simulink model "EMC_no_gaze"  (R2015a)
settings: Solver=ode4  SolverMode=MultiTasking  StartTime=0.0  StopTime=inf  FixedStep=BKIN_STEP_TIME  RelTol=1e-3
StartFcn:
  |  warndlg('Dexterit-E models cannot run under simulation. Please compile your model and run it from within Dexterit-E.');set_param(bdroot,'SimulationCommand','stop')
model workspace (MAT data in the model file):
  BKIN_KINEMATIC_FRAME_SIZE = 400
  BKIN_STEP_TIME = 0.00025
  COLOR = 4
  COL_X = 1
  COL_Y = 2
  E_NO_EVENT = 0
  LOAD_X = 1
  LOAD_Y = 2
  MOVEMENT_DELAY = 3
  PATH_LENGTH = 1
  PATH_PERIOD = 2
  POST_TRIAL_DELAY = 4
  RADIUS = 3
  TRAJECTORY = 1
  TRAJECTORY_TYPE = 2
  TRIAL_END = 3
  TRIAL_MOVEMENT = 2
  TRIAL_RESET = 4
  TRIAL_START = 1
  X_POSITION = 1
  Y_POSITION = 2
  col_x = 1
  col_y = 2
  ANGULAR_THRESHOLD = 5
  GAZE_EXIT = 6
  START_REACHED = 7
  FIXATION_DURATION = 6
  TRACKING_TARGET_ROW = 7
  FEEDBACK_COLOR = 5
  CROSS_LOGICAL_RADIUS = 8
  DETECT_FIXATION = 8
  GAZE_IN_TARGET = 5
  START_STABILIZATION = 9
  HAND_IN_TARGET = 9
  BACKGROUND_LOAD = 10
  DIST_BETWEEN_TRAJ = 11
libraries: simulink x14, xpcrtudplib x12, xpcutilitieslib x10, xpcobsoletelib x8, ethercat x2, General x2, Video x2, KINARM_EP_loads x1, KINARM_general x1
(part 2 of 7)

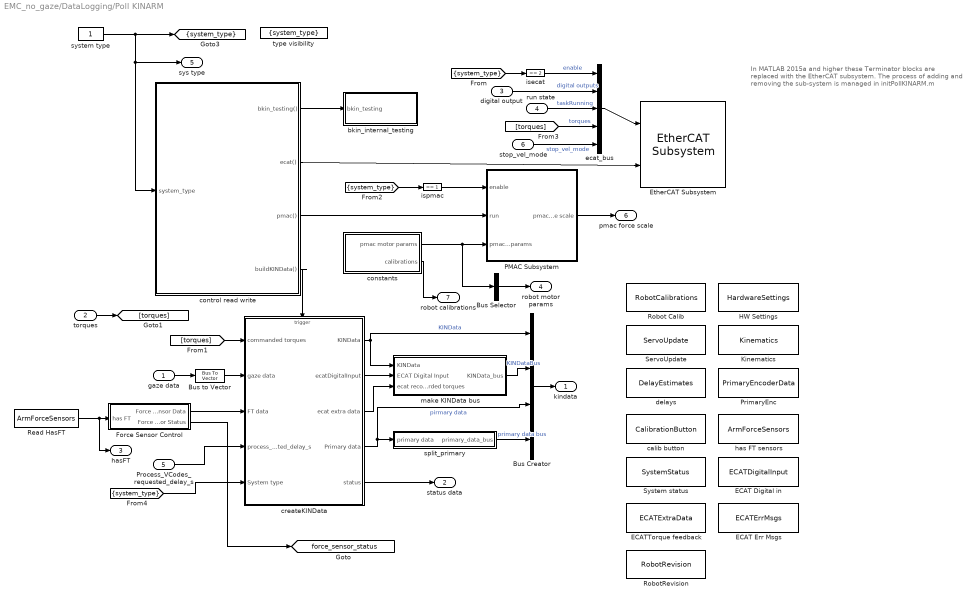
== system EMC_no_gaze/DataLogging/Poll KINARM ==
  note: In MATLAB 2015a and higher these Terminator blocks
      | are replaced with the EtherCAT subsystem. The process of
      | adding and removing the sub-system is managed in
      | initPollKINARM.m
  gaze data : Inport
  torques : Inport  Port=2
  digital output : Inport  Port=3
  run state : Inport  Port=4
  Process_VCodes_requested_delay_s : Inport  Port=5
  stop_vel_mode : Inport  Port=6
  Bus Creator : BusCreator
  Bus Selector : BusSelector  OutputSignals=robot1MotorParams,robot2MotorParams  OutputAsBus=on
  Bus to Vector : BusToVector
  ECAT Digital in : DataStoreMemory  DataStoreName=ECATDigitalInput  ReadBeforeWriteMsg=error  WriteAfterWriteMsg=warning  WriteAfterReadMsg=error  InitialValue=[0, 0, 0, 0, 0, 0, 0, 0]  OutDataTypeStr=uint32
  ECAT Err Msgs : DataStoreMemory  DataStoreName=ECATErrMsgs  ReadBeforeWriteMsg=error  WriteAfterWriteMsg=warning  WriteAfterReadMsg=error  InitialValue=zeros(4, 5)  OutDataTypeStr=double
  ECATTorque feedback : DataStoreMemory  DataStoreName=ECATExtraData  ReadBeforeWriteMsg=error  WriteAfterWriteMsg=warning  WriteAfterReadMsg=error  InitialValue=[0, 0, 0, 0, 0, 0, 0, 0, 0, 0]  OutDataTypeStr=double
  EtherCAT Subsystem : ethercat/EtherCAT Subsystem  SystemSampleTime=BKIN_STEP_TIME
  Force Sensor Control : Subsystem  TreatAsAtomicUnit=on
      settings: RTWSystemCode=Nonreusable function  RTWFileNameOpts=Use function name
  HW Settings : DataStoreMemory  DataStoreName=HardwareSettings  ReadBeforeWriteMsg=error  WriteAfterWriteMsg=warning  WriteAfterReadMsg=error  InitialValue=zeros(24, 1)  OutDataTypeStr=double
  Kinematics : DataStoreMemory  DataStoreName=Kinematics  ReadBeforeWriteMsg=error  WriteAfterWriteMsg=warning  WriteAfterReadMsg=error  InitialValue=zeros(20, 1)  OutDataTypeStr=double
  PMAC Subsystem : Subsystem
      settings: RTWSystemCode=Nonreusable function  RTWFileNameOpts=Use function name
  PrimaryEnc : DataStoreMemory  DataStoreName=PrimaryEncoderData  ReadBeforeWriteMsg=error  WriteAfterWriteMsg=warning  WriteAfterReadMsg=error  InitialValue=zeros(12, 1)  OutDataTypeStr=double
  Read HasFT : DataStoreRead  DataStoreName=ArmForceSensors  SampleTime=BKIN_STEP_TIME
  Robot Calib : DataStoreMemory  DataStoreName=RobotCalibrations  InitialValue=zeros(16, 1)  OutDataTypeStr=double
  RobotRevision : DataStoreMemory  DataStoreName=RobotRevision  ReadBeforeWriteMsg=error  WriteAfterWriteMsg=warning  WriteAfterReadMsg=error  InitialValue=[1, 1]  OutDataTypeStr=double
  ServoUpdate : DataStoreMemory  DataStoreName=ServoUpdate  ReadBeforeWriteMsg=error  WriteAfterWriteMsg=warning  WriteAfterReadMsg=error  OutDataTypeStr=uint32
  System status : DataStoreMemory  DataStoreName=SystemStatus  ReadBeforeWriteMsg=error  WriteAfterWriteMsg=warning  WriteAfterReadMsg=error  InitialValue=zeros(1, 7)  OutDataTypeStr=uint32
  bkin_internal_testing : Subsystem
  calib button : DataStoreMemory  DataStoreName=CalibrationButton  ReadBeforeWriteMsg=error  WriteAfterWriteMsg=warning  WriteAfterReadMsg=error  OutDataTypeStr=uint32
  constants : Subsystem
      settings: RTWSystemCode=Nonreusable function  RTWFileNameOpts=Use function name
  control read write : Stateflow chart  TreatAsAtomicUnit=on
  createKINData : Subsystem
      settings: RTWSystemCode=Nonreusable function  RTWFileNameOpts=Use function name
  delays : DataStoreMemory  DataStoreName=DelayEstimates  ReadBeforeWriteMsg=error  WriteAfterWriteMsg=warning  WriteAfterReadMsg=error  InitialValue=zeros(4, 1)  OutDataTypeStr=double
  ecat_bus : BusCreator  Inputs=5
  has FT sensors : DataStoreMemory  DataStoreName=ArmForceSensors  InitialValue=[0, 0]  OutDataTypeStr=double
  isecat : simulink/Logic and Bit Operations/Compare To Constant  relop===  const=2  OutDataTypeStr=boolean
  ispmac : simulink/Logic and Bit Operations/Compare To Constant  relop===  const=1  OutDataTypeStr=boolean
  make KINData bus : Subsystem
  split_primary : Subsystem
  system type : Constant
  type visibility : GotoTagVisibility  GotoTag=system_type
  kindata : Outport
  status data : Outport  Port=2
  hasFT : Outport  Port=3
  robot motor params : Outport  Port=4
  sys type : Outport  Port=5
  pmac force scale : Outport  Port=6
  robot calibrations : Outport  Port=7
  tag scope: force_sensor_status=global, system_type=scoped
  wires:
  control read write/2(ecat()) -> EtherCAT Subsystem/2
  ecat_bus/1 -> EtherCAT Subsystem/1
  stop_vel_mode/1 -> ecat_bus/5  "stop_vel_mode"
  Bus Selector/1 -> robot motor params/1
  Bus Creator/1 -> kindata/1
  Bus to Vector/1 -> createKINData/2(gaze data)
  constants/1(pmac motor params) -> Bus Selector/1, PMAC Subsystem/3(pmac robot params)
  createKINData/1(KINData) -> Bus Creator/1, make KINData bus/1(KINData)  "KINData"
  createKINData/4(Primary data) -> Bus Creator/3, split_primary/1(primary data)  "pirmary data"
  createKINData/5(status) -> status data/1
  gaze data/1 -> Bus to Vector/1
  Force Sensor Control/1(Force Sensor Data) -> createKINData/3(FT data)
  system type/1 -> [system_type], control read write/1(system_type), sys type/1
  control read write/1(bkin_testing()) -> bkin_internal_testing/1(bkin_testing)
  control read write/3(pmac()) -> PMAC Subsystem/2(run)
  control read write/4(buildKINData()) -> createKINData/Trigger
  [system_type] -> isecat/1
  [system_type] -> ispmac/1
  ispmac/1 -> PMAC Subsystem/1(enable)
  Read HasFT/1 -> hasFT/1, Force Sensor Control/1(has FT)
  make KINData bus/1(KINData_bus) -> Bus Creator/2  "KINDataBus"
  split_primary/1(primary_data_bus) -> Bus Creator/4  "primary data bus"
  PMAC Subsystem/1(pmac force scale) -> pmac force scale/1
  constants/2(calibrations) -> robot calibrations/1
  createKINData/2(ecatDigitalInput) -> make KINData bus/2(ECAT Digital Input)
  digital output/1 -> ecat_bus/2  "digital outputs"
  run state/1 -> ecat_bus/3  "taskRunning"
  isecat/1 -> ecat_bus/1  "enable"
  torques/1 -> [torques]
  [torques] -> createKINData/1(commanded torques)
  [torques] -> ecat_bus/4  "torques"
  createKINData/3(ecat extra data) -> make KINData bus/3(ecat recorded torques)
  Process_VCodes_requested_delay_s/1 -> createKINData/4(process_vcodes_requested_delay_s)
  Force Sensor Control/2(Force Sensor Status) -> [force_sensor_status]
  [system_type] -> createKINData/5(System type)

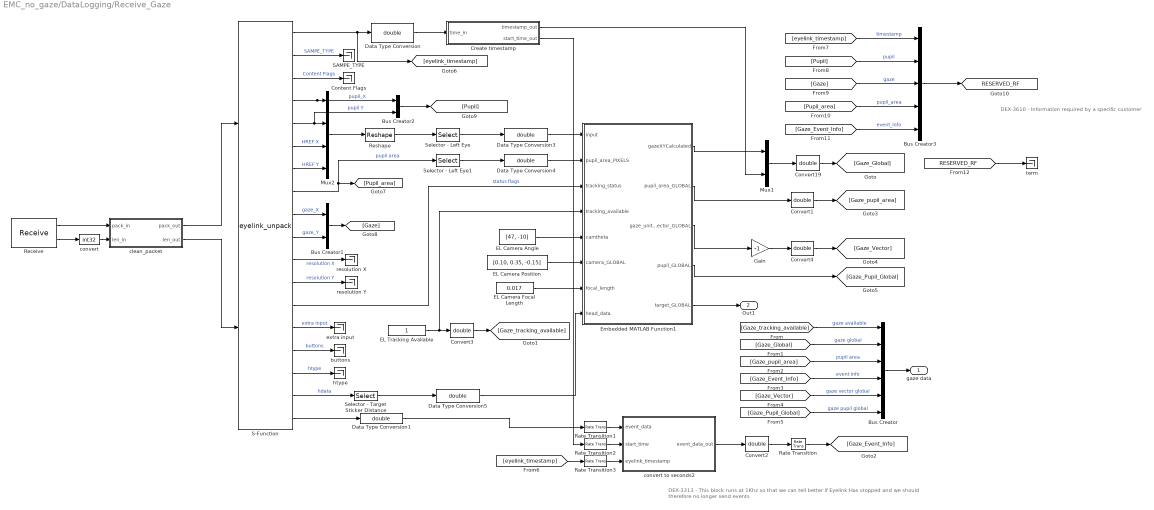
== system EMC_no_gaze/DataLogging/Receive_Gaze ==
  note: DEX-3610 - Information required by a specific customer
  note: DEX-3313 - This block runs at 1Khz so that we can tell better if Eyelink
      | Has stopped and we should therefore no longer send events
  Bus Creator : BusCreator  Inputs=6
  Bus Creator1 : BusCreator  Inputs=2
  Bus Creator2 : BusCreator  Inputs=2
  Bus Creator3 : BusCreator  Inputs=5
  Content Flags : Terminator
  Convert{1..4,19} (5 alike) : DataTypeConversion  OutDataTypeStr=double
  Create timestamp : MATLAB Function  TreatAsAtomicUnit=on
  Data Type Conversion{,1,3..5} (5 alike) : DataTypeConversion  OutDataTypeStr=double
  EL Camera Angle : Constant  Value=[47, -10]  VectorParams1D=off  OutDataTypeStr=double
  EL Camera Focal Length : Constant  Value=0.017  VectorParams1D=off  OutDataTypeStr=double
  EL Camera Position : Constant  Value=[0.10, 0.35, -0.15]  VectorParams1D=off  OutDataTypeStr=double
  EL Tracking Available : Constant  VectorParams1D=off  OutDataTypeStr=double
  Embedded MATLAB Function1 : MATLAB Function  TreatAsAtomicUnit=on
  Gain : Gain  Gain=-1
  Mux1 : Mux  Inputs=2
  Mux2 : Mux
  Rate Transition{,1..3} (4 alike) : RateTransition  Integrity=off
  Receive : xpcrtudplib/Legacy UDP/Receive   ipAddress=0.0.0.0  ipPort=4000  width=512  vblLen=on  sampletime=BKIN_STEP_TIME
  Reshape : Reshape  OutputDimensionality=Customize  OutputDimensions=[2,4]
  S-Function : S-Function  FunctionName=eyelink_unpack
  SAMPE_TYPE : Terminator
  Selector - Left Eye : Selector  NumberOfDimensions=2  InputPortWidth=3  IndexOptions=Index vector (dialog),Index vector (dialog)  Indices=1,-1  OutputSizes=1,1
  Selector - Left Eye1 : Selector
  Selector - Target Sticker Distance : Selector  Indices=1:3
  buttons : Terminator
  clean_packet : MATLAB Function  TreatAsAtomicUnit=on
  convert : DataTypeConversion  OutDataTypeStr=int32
  convert to seconds2 : MATLAB Function  TreatAsAtomicUnit=on  SystemSampleTime=0.001
  extra input : Terminator
  htype : Terminator
  resolution X : Terminator
  resolution Y : Terminator
  term : Terminator
  gaze data : Outport
  Out1 : Outport  Port=2
  tag scope: RESERVED_RF=global
  wires:
  Rate Transition3/1 -> convert to seconds2/3(eyelink_timestamp)
  Rate Transition2/1 -> convert to seconds2/2(start_time)
  Rate Transition1/1 -> convert to seconds2/1(event_data)
  [Gaze_Pupil_Global] -> Bus Creator/6  "gaze pupil global"
  Embedded MATLAB Function1/4(pupil_GLOBAL) -> [Gaze_Pupil_Global]
  Gain/1 -> Convert4/1
  Bus Creator/1 -> gaze data/1
  [Gaze_Event_Info] -> Bus Creator/4  "event info"
  [Gaze_pupil_area] -> Bus Creator/3  "pupil area"
  [Gaze_Global] -> Bus Creator/2  "gaze global"
  [Gaze_tracking_available] -> Bus Creator/1  "gaze available"
  EL Tracking Available/1 -> Embedded MATLAB Function1/4(tracking_available), Convert3/1
  EL Camera Position/1 -> Embedded MATLAB Function1/6(camera_GLOBAL)
  EL Camera Angle/1 -> Embedded MATLAB Function1/5(camtheta)
  Selector - Target Sticker Distance/1 -> Data Type Conversion5/1
  Selector - Left Eye/1 -> Data Type Conversion3/1
  Reshape/1 -> Selector - Left Eye/1
  Mux2/1 -> Reshape/1
  S-Function/7 -> Mux2/4  "HREF Y"
  S-Function/6 -> Mux2/3  "HREF X"
  S-Function/5 -> Bus Creator2/2, Mux2/2  "pupil Y"
  S-Function/4 -> Bus Creator2/1, Mux2/1  "pupil_X"
  Receive/2 -> convert/1
  S-Function/17 -> Selector - Target Sticker Distance/1  "hdata"
  S-Function/16 -> htype/1  "htype"
  S-Function/15 -> buttons/1  "buttons"
  S-Function/14 -> extra input/1  "extra input"
  S-Function/13 -> Embedded MATLAB Function1/3(tracking_status)  "status flags"
  S-Function/12 -> resolution Y/1  "resolution Y"
  S-Function/11 -> resolution X/1  "resolution X"
  S-Function/8 -> Selector - Left Eye1/1, [Pupil_area]  "pupil area"
  S-Function/3 -> Content Flags/1  "Content Flags"
  S-Function/2 -> SAMPE_TYPE/1  "SAMPE_TYPE"
  S-Function/9 -> Bus Creator1/1  "gaze_X"
  S-Function/10 -> Bus Creator1/2  "gaze_Y"
  Mux1/1 -> Convert19/1
  Embedded MATLAB Function1/1(gazeXYCalculated) -> Mux1/1
  Data Type Conversion/1 -> Create timestamp/1(time_in)
  S-Function/1 -> [eyelink_timestamp], Data Type Conversion/1
  S-Function/18 -> Data Type Conversion1/1
  Data Type Conversion1/1 -> Rate Transition1/1
  convert to seconds2/1(event_data_out) -> Convert2/1
  Create timestamp/2(start_time_out) -> Rate Transition2/1
  Data Type Conversion3/1 -> Embedded MATLAB Function1/1(input)
  Data Type Conversion5/1 -> Embedded MATLAB Function1/8(head_data)
  Embedded MATLAB Function1/2(pupil_area_GLOBAL) -> Convert1/1
  Data Type Conversion4/1 -> Embedded MATLAB Function1/2(pupil_area_PIXELS)
  EL Camera Focal Length/1 -> Embedded MATLAB Function1/7(focal_length)
  Selector - Left Eye1/1 -> Data Type Conversion4/1
  Receive/1 -> clean_packet/1(pack_in)
  convert/1 -> clean_packet/2(len_in)
  clean_packet/1(pack_out) -> S-Function/1
  clean_packet/2(len_out) -> S-Function/2
  Convert19/1 -> [Gaze_Global]
  Convert1/1 -> [Gaze_pupil_area]
  Convert2/1 -> Rate Transition/1
  Convert3/1 -> [Gaze_tracking_available]
  Convert4/1 -> [Gaze_Vector]
  Embedded MATLAB Function1/3(gaze_unit_vector_GLOBAL) -> Gain/1
  [Gaze_Vector] -> Bus Creator/5  "gaze vector global"
  Create timestamp/1(timestamp_out) -> Mux1/2
  Rate Transition/1 -> [Gaze_Event_Info]
  [eyelink_timestamp] -> Rate Transition3/1
  Bus Creator1/1 -> [Gaze]
  Bus Creator2/1 -> [Pupil]
  [Gaze_Event_Info] -> Bus Creator3/5  "event_info"
  [Pupil_area] -> Bus Creator3/4  "pupil_area"
  [Gaze] -> Bus Creator3/3  "gaze"
  [Pupil] -> Bus Creator3/2  "pupil"
  [eyelink_timestamp] -> Bus Creator3/1  "timestamp"
  Bus Creator3/1 -> [RESERVED_RF]
  [RESERVED_RF] -> term/1
  Embedded MATLAB Function1/5(target_GLOBAL) -> Out1/1

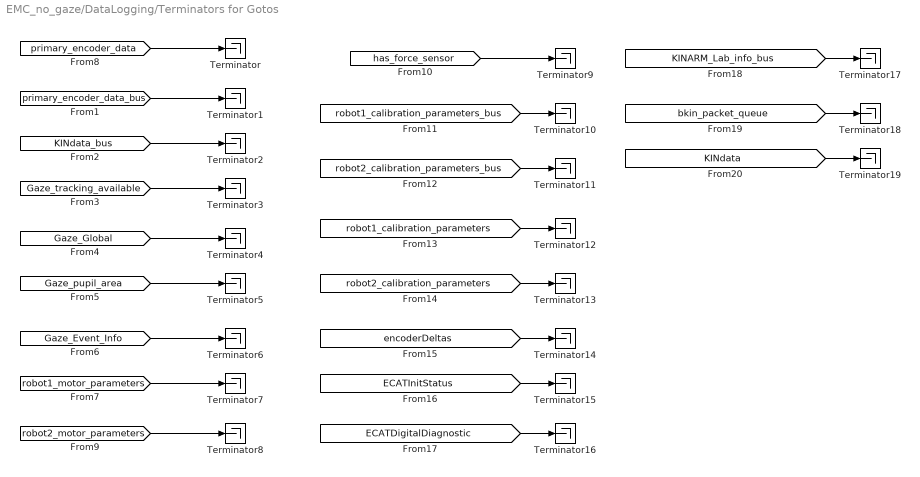
== system EMC_no_gaze/DataLogging/Terminators for Gotos ==
  Terminator{,1..19} (20 alike) : Terminator
  wires:
  [has_force_sensor] -> Terminator9/1
  [robot2_motor_parameters] -> Terminator8/1
  [robot1_motor_parameters] -> Terminator7/1
  [Gaze_Event_Info] -> Terminator6/1
  [Gaze_pupil_area] -> Terminator5/1
  [Gaze_Global] -> Terminator4/1
  [Gaze_tracking_available] -> Terminator3/1
  [KINdata_bus] -> Terminator2/1
  [primary_encoder_data_bus] -> Terminator1/1
  [primary_encoder_data] -> Terminator/1
  [robot1_calibration_parameters_bus] -> Terminator10/1
  [robot2_calibration_parameters_bus] -> Terminator11/1
  [robot1_calibration_parameters] -> Terminator12/1
  [robot2_calibration_parameters] -> Terminator13/1
  [encoderDeltas] -> Terminator14/1
  [ECATInitStatus] -> Terminator15/1
  [ECATDigitalDiagnostic] -> Terminator16/1
  [KINARM_Lab_info_bus] -> Terminator17/1
  [bkin_packet_queue] -> Terminator18/1
  [KINdata] -> Terminator19/1

== system EMC_no_gaze/DataLogging/apply loads ==
  system_type : Inport
  torques : Inport  Port=2
  pmac force scale : Inport  Port=3
  motor params : Inport  Port=4
  Bus Selector3 : BusSelector  OutputSignals=robot1MotorParams,robot2MotorParams
  EtherCAT Apply Loads : ethercat/ECAT Apply Loads
  apply pmac loads : Subsystem
      settings: RTWSystemCode=Nonreusable function  RTWFileNameOpts=Use function name
  isecat : simulink/Logic and Bit Operations/Compare To Constant  relop===  const=2  OutDataTypeStr=boolean
  isecat1 : simulink/Logic and Bit Operations/Compare To Constant  relop===  const=1  OutDataTypeStr=boolean
  verify NaN : MATLAB Function  TreatAsAtomicUnit=on
  wires:
  [torques] -> EtherCAT Apply Loads/1
  isecat/1 -> EtherCAT Apply Loads/Enable
  Bus Selector3/2 -> apply pmac loads/4(Robot 2 motor parms)  "<robot2MotorParams>"
  Bus Selector3/1 -> apply pmac loads/3(Robot 1 motor parms)  "<robot1MotorParams>"
  pmac force scale/1 -> apply pmac loads/1(Force scale)
  motor params/1 -> Bus Selector3/1
  [system_type] -> isecat1/1
  isecat1/1 -> apply pmac loads/Enable
  [system_type] -> isecat/1
  torques/1 -> verify NaN/1(torques_in)
  [torques] -> apply pmac loads/2(Torques)
  system_type/1 -> [system_type]
  verify NaN/1(torques_out) -> [torques]

== system EMC_no_gaze/DataLogging/compare encoders ==
  Bus Selector4 : BusSelector  OutputSignals=Robot1.a1_link_angles,Robot2.a2_link_angles
  Bus Selector5 : BusSelector  OutputSignals=robot1.a1_link_angles,robot2.a2_link_angles
  Mux : Mux  Inputs=2
  Mux1 : Mux  Inputs=2
  delta : MATLAB Function  TreatAsAtomicUnit=on
  encoder deltas : Outport
  wires:
  [KINdata_bus] -> Bus Selector4/1
  [primary_encoder_data_bus] -> Bus Selector5/1
  Bus Selector4/1 -> Mux/1  "<a1_link_angles>"
  Bus Selector4/2 -> Mux/2  "<a2_link_angles>"
  Bus Selector5/1 -> Mux1/1  "<a1_link_angles>"
  Bus Selector5/2 -> Mux1/2  "<a2_link_angles>"
  Mux/1 -> delta/1(secondaryEncAngles)
  Mux1/1 -> delta/2(primaryEncAngles)
  delta/1(deltas) -> encoder deltas/1

== system EMC_no_gaze/DataLogging/create_lab_info ==
  Bus Creator3 : BusCreator  Inputs=7
  Subsystem : Subsystem
  arm_count : Constant  Value=0
  fp1_present : Constant  Value=0
  fp2_present : Constant  Value=0
  gaze_tracker_present : Constant  Value=0
  robot_lift_present : Constant  Value=0
  tag scope: KINARM_Lab_info_bus=global
  wires:
  fp1_present/1 -> Bus Creator3/5  "has_force_plate_1"
  Bus Creator3/1 -> [KINARM_Lab_info_bus]
  Subsystem/2(robot_2_info) -> Bus Creator3/3  "robot_2"
  Subsystem/1(robot_1_info) -> Bus Creator3/2  "robot_1"
  robot_lift_present/1 -> Bus Creator3/7  "has_robot_lift"
  gaze_tracker_present/1 -> Bus Creator3/4  "has_gaze_tracker"
  arm_count/1 -> Bus Creator3/1  "robot_count"
  fp2_present/1 -> Bus Creator3/6  "has_force_plate_2"

== system EMC_no_gaze/DataLogging/gaze gotos ==
  In1 : Inport
  Bus Selector : BusSelector  OutputSignals=gaze available,gaze global,pupil area,event info,gaze vector global,gaze pupil global
  tag scope: Gaze_Event_Info=global, Gaze_Global=global, Gaze_Pupil_Global=global, Gaze_Vector_Global=global, Gaze_pupil_area=global, Gaze_tracking_available=global
  wires:
  Bus Selector/5 -> [Gaze_Vector_Global]  "<gaze vector global>"
  Bus Selector/6 -> [Gaze_Pupil_Global]  "<gaze pupil global>"
  Bus Selector/4 -> [Gaze_Event_Info]  "<event info>"
  Bus Selector/3 -> [Gaze_pupil_area]  "<pupil area>"
  Bus Selector/2 -> [Gaze_Global]  "<gaze global>"
  Bus Selector/1 -> [Gaze_tracking_available]  "<gaze available>"
  In1/1 -> Bus Selector/1

== system EMC_no_gaze/DataLogging/kindata gotos ==
  In1 : Inport
  Bus Selector1 : BusSelector  OutputSignals=KINData,KINDataBus,pirmary data,primary data bus
  tag scope: KINdata=global, KINdata_bus=global, primary_encoder_data=global, primary_encoder_data_bus=global
  wires:
  Bus Selector1/4 -> [primary_encoder_data_bus]  "<primary data bus>"
  Bus Selector1/3 -> [primary_encoder_data]  "<pirmary data>"
  Bus Selector1/2 -> [KINdata_bus]  "<KINDataBus>"
  Bus Selector1/1 -> [KINdata]  "<KINData>"
  In1/1 -> Bus Selector1/1

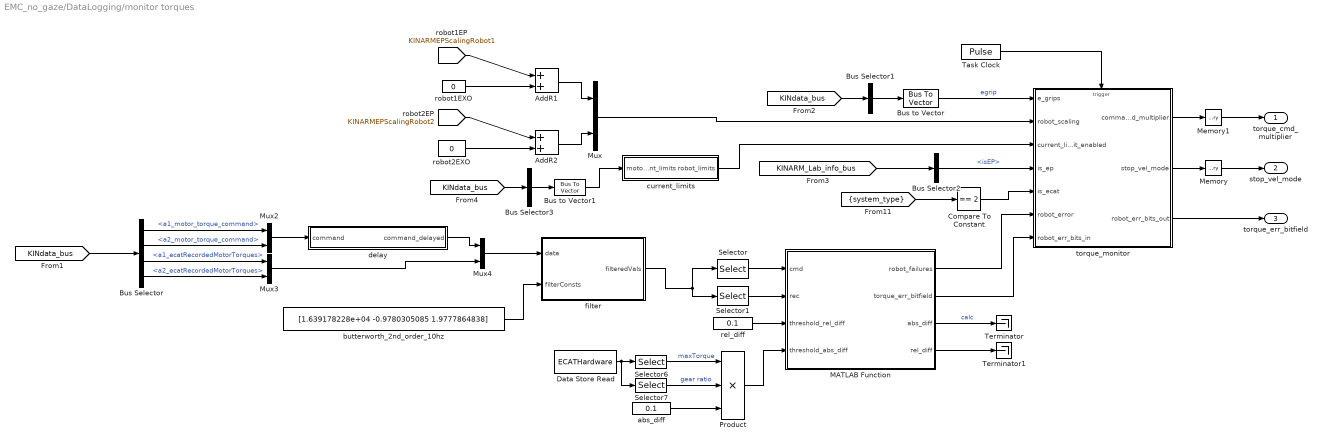
== system EMC_no_gaze/DataLogging/monitor torques ==
  AddR1 : Sum
  AddR2 : Sum
  Bus Selector : BusSelector  OutputSignals=Robot1.a1_motor_torque_command,Robot2.a2_motor_torque_command,Robot1.a1_ecatRecordedMotorTorques,Robot2.a2_ecatRecordedMotorTorques
  Bus Selector1 : BusSelector  OutputSignals=Robot1.a1_ep_grip_sensor,Robot2.a2_ep_grip_sensor  OutputAsBus=on
  Bus Selector2 : BusSelector  OutputSignals=robot_1.isEP
  Bus Selector3 : BusSelector  OutputSignals=Robot1.a1_ecatCurrentLimitEnabled,Robot2.a2_ecatCurrentLimitEnabled  OutputAsBus=on
  Bus to Vector : BusToVector
  Bus to Vector1 : BusToVector
  Compare To Constant : simulink/Logic and Bit Operations/Compare To Constant  relop===  const=2  OutDataTypeStr=boolean
  Data Store Read : DataStoreRead  DataStoreName=ECATHardware  SampleTime=BKIN_STEP_TIME
  MATLAB Function : MATLAB Function  TreatAsAtomicUnit=on
  Memory : Memory
  Memory1 : Memory
  Mux{,2..4} (4 alike) : Mux  Inputs=2
  Product : Product  Inputs=3
  Selector : Selector  Indices=[1:4]
  Selector1 : Selector  Indices=[5:8]
  Selector6 : Selector  Indices=[1:4]
  Selector7 : Selector  Indices=[5:8]
  Task Clock : DiscretePulseGenerator  PulseType=Time based  Period=.001  PulseWidth=50  SampleTime=0.0005
  Terminator : Terminator
  Terminator1 : Terminator
  abs_diff : Constant  Value=0.1
  butterworth_2nd_order_10hz : Constant  Value=[1.639178228e+04 -0.9780305085 1.9777864838]
  current_limits : MATLAB Function  TreatAsAtomicUnit=on  SystemSampleTime=BKIN_STEP_TIME
  delay : Subsystem
  filter : MATLAB Function  TreatAsAtomicUnit=on  SystemSampleTime=BKIN_STEP_TIME
  rel_diff : Constant  Value=0.1
  robot1EXO : Constant  Value=0
  robot2EXO : Constant  Value=0
  torque_monitor : Stateflow chart  TreatAsAtomicUnit=on
  torque_cmd_multiplier : Outport
  stop_vel_mode : Outport  Port=2
  torque_err_bitfield : Outport  Port=3
  wires:
  MATLAB Function/4(rel_diff) -> Terminator1/1
  MATLAB Function/3(abs_diff) -> Terminator/1  "calc"
  butterworth_2nd_order_10hz/1 -> filter/2(filterConsts)
  Mux4/1 -> filter/1(data)
  Memory/1 -> stop_vel_mode/1
  Memory1/1 -> torque_cmd_multiplier/1
  Bus Selector2/1 -> torque_monitor/4(is_ep)  "<isEP>"
  [system_type] -> Compare To Constant/1
  [KINARM_Lab_info_bus] -> Bus Selector2/1
  Bus to Vector/1 -> torque_monitor/1(e_grips)  "egrip"
  Bus Selector1/1 -> Bus to Vector/1
  [KINdata_bus] -> Bus Selector1/1
  MATLAB Function/1(robot_failures) -> torque_monitor/6(robot_error)
  Selector1/1 -> MATLAB Function/2(rec)
  Selector/1 -> MATLAB Function/1(cmd)
  filter/1(filteredVals) -> Selector/1, Selector1/1
  Mux3/1 -> Mux4/2
  delay/1(command_delayed) -> Mux4/1
  Mux2/1 -> delay/1(command)
  Bus Selector/3 -> Mux3/1  "<a1_ecatRecordedMotorTorques>"
  Bus Selector/4 -> Mux3/2  "<a2_ecatRecordedMotorTorques>"
  Bus Selector/2 -> Mux2/2  "<a2_motor_torque_command>"
  Bus Selector/1 -> Mux2/1  "<a1_motor_torque_command>"
  [KINdata_bus] -> Bus Selector/1
  Compare To Constant/1 -> torque_monitor/5(is_ecat)
  Task Clock/1 -> torque_monitor/Trigger
  torque_monitor/2(stop_vel_mode) -> Memory/1
  torque_monitor/1(command_multiplier) -> Memory1/1
  [KINdata_bus] -> Bus Selector3/1
  AddR1/1 -> Mux/1
  AddR2/1 -> Mux/2
  Bus Selector3/1 -> Bus to Vector1/1
  Mux/1 -> torque_monitor/2(robot_scaling)
  MATLAB Function/2(torque_err_bitfield) -> torque_monitor/7(robot_err_bits_in)
  torque_monitor/3(robot_err_bits_out) -> torque_err_bitfield/1
  Data Store Read/1 -> Selector7/1, Selector6/1
  Selector6/1 -> Product/1  "maxTorque"
  Product/1 -> MATLAB Function/4(threshold_abs_diff)
  Selector7/1 -> Product/2  "gear ratio"
  abs_diff/1 -> Product/3
  rel_diff/1 -> MATLAB Function/3(threshold_rel_diff)
  current_limits/1(robot_limits) -> torque_monitor/3(current_limit_enabled)
  Bus to Vector1/1 -> current_limits/1(motor_current_limits)
  robot1EXO/1 -> AddR1/2
  robot2EXO/1 -> AddR2/2
  [KINARMEPScalingRobot1] -> AddR1/1
  [KINARMEPScalingRobot2] -> AddR2/1

== system EMC_no_gaze/DataLogging/motor gotos ==
  In1 : Inport
  Bus Selector2 : BusSelector  OutputSignals=robot1MotorParams,robot2MotorParams
  tag scope: robot1_motor_parameters=global, robot2_motor_parameters=global
  wires:
  Bus Selector2/2 -> [robot2_motor_parameters]  "<robot2MotorParams>"
  Bus Selector2/1 -> [robot1_motor_parameters]  "<robot1MotorParams>"
  In1/1 -> Bus Selector2/1

== system EMC_no_gaze/DataLogging/robot gotos ==
  In1 : Inport
  Bus Selector3 : BusSelector  OutputSignals=robot1 calibration params,robot2 calibration params
  Bus to Vector : BusToVector
  Bus to Vector1 : BusToVector
  tag scope: robot1_calibration_parameters=global, robot1_calibration_parameters_bus=global, robot2_calibration_parameters=global, robot2_calibration_parameters_bus=global
  wires:
  Bus Selector3/1 -> [robot1_calibration_parameters_bus], Bus to Vector/1  "<robot1 calibration params>"
  Bus Selector3/2 -> [robot2_calibration_parameters_bus], Bus to Vector1/1  "<robot2 calibration params>"
  Bus to Vector/1 -> [robot1_calibration_parameters]
  Bus to Vector1/1 -> [robot2_calibration_parameters]
  In1/1 -> Bus Selector3/1

== system EMC_no_gaze/KINARM_EP_Apply_Loads/detect motor state ==
  Bus Selector1 : BusSelector  OutputSignals=R1Info.isECAT
  Bus Selector2 : BusSelector  OutputSignals=Robot1.a1_motor_status,Robot1.a1_ep_grip_sensor
  MATLAB Function : MATLAB Function  TreatAsAtomicUnit=on
  motors enabled : Outport
  wires:
  Bus Selector2/2 -> MATLAB Function/2(grip_sensor)  "<a1_ep_grip_sensor>"
  [robot1_motor_parameters] -> Bus Selector1/1
  Bus Selector2/1 -> MATLAB Function/1(motor_status)  "<a1_motor_status>"
  [KINdata_bus] -> Bus Selector2/1
  Bus Selector1/1 -> MATLAB Function/3(is_ecat)  "<isECAT>"
  MATLAB Function/1(motors_enabled) -> motors enabled/1

== system EMC_no_gaze/KINARM_EP_Apply_Loads/detect motor state1 ==
  Bus Selector1 : BusSelector  OutputSignals=R2Info.isECAT
  Bus Selector2 : BusSelector  OutputSignals=Robot2.a2_motor_status,Robot2.a2_ep_grip_sensor
  MATLAB Function : MATLAB Function  TreatAsAtomicUnit=on
  motors enabled : Outport
  wires:
  Bus Selector2/2 -> MATLAB Function/2(grip_sensor)  "<a2_ep_grip_sensor>"
  [robot2_motor_parameters] -> Bus Selector1/1
  Bus Selector2/1 -> MATLAB Function/1(motor_status)  "<a2_motor_status>"
  [KINdata_bus] -> Bus Selector2/1
  Bus Selector1/1 -> MATLAB Function/3(is_ecat)  "<isECAT>"
  MATLAB Function/1(motors_enabled) -> motors enabled/1

== system EMC_no_gaze/DataLogging/Create KINARM Data Subsystem/gaze_data ==
  Mux : Mux  Inputs=5
  gaze_channels : Outport
  wires:
  [Gaze_Global] -> Mux/1
  Mux/1 -> gaze_channels/1
  [Gaze_pupil_area] -> Mux/2
  [Gaze_Vector_Global] -> Mux/3
  [Gaze_Event_Info] -> Mux/5
  [Gaze_Pupil_Global] -> Mux/4

== system EMC_no_gaze/DataLogging/Create KINARM Data Subsystem/select KINData ==
  Bus Selector : BusSelector  OutputSignals=Robot1.a1_link_angles,Robot1.a1_link_velocities,Robot1.a1_link_accelerations,Robot1.a1_hand_position,Robot1.a1_motor_torque_command,Robot1.a1_force_sensor_force_xyz,Robot1.a1_force_sensor_torque_xyz,Robot1.a1_force_sensor_timestamp,Robot1.a1_ecatRecordedMotorTorques,Robot2.a2_link_angles,Robot2.a2_link_velocities,Robot2.a2_link_accelerations,Robot2.a2_hand_position,Robot2.a2_motor_torque_command,Robot2.a2_force_sensor_force_xyz,Robot2.a2_force_sensor_torque_xyz,Robot2.a2_force_sensor_timestamp,Robot2.a2_ecatRecordedMotorTorques,Robot1.a1_force_sensor_status,Robot2.a2_force_sensor_status
  Demux : Demux  Outputs=2
  MATLAB Function : MATLAB Function  TreatAsAtomicUnit=on
  Mux : Mux  Inputs=8
  Mux1 : Mux  Inputs=9
  Mux2 : Mux  Inputs=5
  Mux3 : Mux  Inputs=2
  Out1 : Outport
  wires:
  [KINdata_bus] -> Bus Selector/1
  Bus Selector/1 -> Mux/1  "<a1_link_angles>"
  Bus Selector/2 -> Mux/2  "<a1_link_velocities>"
  Bus Selector/3 -> Mux/3  "<a1_link_accelerations>"
  Bus Selector/4 -> Mux/4  "<a1_hand_position>"
  Bus Selector/5 -> Mux/5  "<a1_motor_torque_command>"
  Bus Selector/6 -> Mux/6  "<a1_force_sensor_force_xyz>"
  Bus Selector/7 -> Mux/7  "<a1_force_sensor_torque_xyz>"
  Bus Selector/8 -> Mux/8  "<a1_force_sensor_timestamp>"
  Bus Selector/9 -> Mux1/1  "<a1_ecatRecordedMotorTorques>"
  Bus Selector/10 -> Mux1/2  "<a2_link_angles>"
  Bus Selector/11 -> Mux1/3  "<a2_link_velocities>"
  Bus Selector/12 -> Mux1/4  "<a2_link_accelerations>"
  Bus Selector/13 -> Mux1/5  "<a2_hand_position>"
  Bus Selector/14 -> Mux1/6  "<a2_motor_torque_command>"
  Bus Selector/15 -> Mux1/7  "<a2_force_sensor_force_xyz>"
  Bus Selector/16 -> Mux1/8  "<a2_force_sensor_torque_xyz>"
  Bus Selector/17 -> Mux1/9  "<a2_force_sensor_timestamp>"
  Bus Selector/18 -> Mux2/5  "<a2_ecatRecordedMotorTorques>"
  Mux2/1 -> Out1/1
  Mux/1 -> Mux2/1
  Mux1/1 -> Mux2/3
  Bus Selector/20 -> Mux3/2  "<a2_force_sensor_status>"
  Bus Selector/19 -> Mux3/1  "<a1_force_sensor_status>"
  Mux3/1 -> MATLAB Function/1(uu)
  MATLAB Function/1(dd_out) -> Demux/1
  Demux/1 -> Mux2/2
  Demux/2 -> Mux2/4

== system EMC_no_gaze/DataLogging/Network Transfer Subsystem/Data Packing Subsystem ==
  note: This index will ensure that we get the correct frames and
      | properly padded with zeros
  note: This subsystem packs data frames to create the data portion of the UDP packets, and sets its strobe output high to indicate when a
      | new chunk of packed data is ready. The number of frames per packet is determined to be the smaller of floor(300/width of signal)
      | and 6, as i) we aim at a maximum size of around 1200 to keep it well below the MTU (300x4 bytes per single), and ii) the hardwired
      | delay structure below stores at most 6 frames before adding empty zeros. A size 300 output is always created, as having an undefined
      | port width causes Simulink problems.
  note: BKIN_KINEMATIC_FRAME_SIZE can be set in performBKINModelSetup.m
      | but you will also need to change value in Send Control Machine in
      | order to make sure the packet size there is also correct.
  data_frame : Inport
  Constant : Constant  Value=zeros(1, BKIN_KINEMATIC_FRAME_SIZE)  OutDataTypeStr=single
  Constant1 : Constant  Value=0
  Counter : Subsystem
  Data Type Conversion : DataTypeConversion  OutDataTypeStr=single  SaturateOnIntegerOverflow=on  RndMeth=Zero
  Ideal Frames Per Packet : Fcn  Expr=floor(BKIN_KINEMATIC_FRAME_SIZE/u(1))
  Math Function : Math  Operator=mod  SaturateOnIntegerOverflow=on
  Max Frames Per Packet : Constant  Value=3
  MinMax : MinMax  Inputs=2
  Mux : Mux
  Product : Product  RndMeth=Zero
  Relational Operator : RelationalOperator  Operator===  OutDataTypeStr=boolean
  Selector : Selector  IndexMode=Zero-based  IndexOptions=Starting index (port)  Indices=[1:300]  OutputSizes=400
  Subtract : Sum  Inputs=+-
  Width : Width
  t-1 : Memory  InheritSampleTime=on
  t-2 : Memory  InheritSampleTime=on
  daq_packet_strobe : Outport
  packed_data : Outport  Port=2
  wires:
  Ideal Frames Per Packet/1 -> MinMax/2
  Width/1 -> Ideal Frames Per Packet/1, Product/1
  Product/1 -> Selector/2
  Subtract/1 -> Product/2
  Max Frames Per Packet/1 -> MinMax/1, Subtract/1
  MinMax/1 -> Subtract/2, Math Function/2
  Constant/1 -> Mux/4
  Selector/1 -> packed_data/1
  Mux/1 -> Selector/1
  Data Type Conversion/1 -> Mux/3, t-1/1
  t-2/1 -> Mux/1
  t-1/1 -> Mux/2, t-2/1
  Math Function/1 -> Relational Operator/2
  Constant1/1 -> Relational Operator/1
  Relational Operator/1 -> daq_packet_strobe/1
  Counter/1(count) -> Math Function/1
  data_frame/1 -> Data Type Conversion/1, Width/1

== system EMC_no_gaze/DataLogging/Network Transfer Subsystem/UDP Receiver ==
  note: At the moment we only care about the ACK packet ID (first element).
      | We have 4 other values we  can return reserved.
  note: DEX-3274: This is the heart of a fix for problems we have found in the UDP sub-system.
      | This code we derrived from the standard UDP receive blocks. The idea here is that the UDP receive
      | block works more-or-less as normal for UDP receive. The main differences are:
      | 1. This version reads the UDP stack twice each time step. This is to look for bad packets and corruption in the UDP stack
      | 2. If this version detects a problem in the UDP stack a call out is made to UDP Receive Port Reset and no more reading is done until the reset is complete.
      |
      | The UDP Receive Port Reset block closes an open UDP port, then reoopens it. This appears to fix any corruption in the UDP stack for the given port.
      | It is critical that this block runs at a relatively slow speed since the reset can take up to 150 micro seconds.
  Trigger UDP reset : Inport
  Data Type Conversion : DataTypeConversion
  Memory1 : Memory  InheritSampleTime=on
  Memory2 : Memory  InheritSampleTime=on
  Rate Transition1 : RateTransition
  Rate Transition2 : RateTransition
  Selector : Selector  Indices=[2:5]
  Terminator{3..7} (5 alike) : Terminator
  UDP Receive : S-Function  FunctionName=BKINUDPReceiveRead  Parameters=ipAdd, ipPort, width, sampletime, vblLen  mask(BKIN UDP Receive Read){ipAddress=999.999.999.999, ipPort=0, width=21, vblLen=off, sampletime=BKIN_STEP_TIME}
      mask prompts: ipAddress "Source IP address:"; ipPort "Local (destination) port:"; width "Output port width (number of bytes):"; vblLen "Allow variable length packets"; sampletime "Sample time:"
      mask help:
      | Modified from legacy UDP Receive block.
      | The rationale for modifying was to enable resetting of the UDP Port while running a model.
      | Because resetting can potentially take longer than one clock cycle, the resetting needed to be split off from the reading to allow them to run at different update rates.
      |
      | Click Help for more details.
      mask init:
      | % BKIN - I tried commenting these out, but it causes build errors.
      | mudp('ipPort', 'IP Port');
      | ipAdd = ipAddressFromString(ipAddress);
      mask Help:
      | Used to read UDP packets. Modified from legacy UDP Read Receive. Must be used with BKIN UDP Receive Port Reset block.
      | 
      | <H2>Description </H2>
      | This block reads a UDP packet from an IP address and port specified in the BKIN UDP Receive Port Reset block.
      | <P>
      | If a packet is read, it will read attempt to read a second packet (i.e. to clear out the queue).
      | <P>
      | If a UDP reset trigger is received, it will coordinate a UDP port reset with the BKIN UDP Receive Port Reset block.
      | During the resetting, UDP reads will not occur.
      |  <P>
      | 
      | <B>UDP Reset Trigger: </B> when this input goes to 1 for at least one clock cycle, it will initiate a reset of the UDP port.
      | <P>
      | <B>Port Info: </B> this vector input must come from the BKIN UDP Receive Port Reset block.
      | <P>
      | <B>Data: </B> This output contains the most recent data read from the UDP packet
      | <P>
      | <B>N: </B> This output contains 1 when a UDP packet was read (or if variable length was checked, the length of the packet).
      | It contains -1 if reads are not allowed (i.e. because the port is being reset).
      | It contains 0 if there was no packet to read.
      | It contains -9 if the length specified in the mask of this block is different that what was specified when the port was opened (i.e. via the BKIN UDP Receive Port Reset block).
      | <P>
      | <B>Data 2: </B> This output contains  the most recent data read from the second read UDP packet (if one was read)
      | <P>
      | <B>N 2: </B> This output contains the same information as the output "N", but for the second UDP packet.
      | <P>
      | <B># double reads: </B> This output contains  the number of times that two UDP packets were read in a single time frame since the start of the task.
      | <P>
      | <B>Request UDP Reset: </B> This output should be connected to UDP Reset input of BKIN UDP Receive Port Reset. It will go to 1 when UDP trigger reset is recieved, and it will stay at 1 until an acknowledgement has been received via Port Info
      | <P>
      | 
      | 
      | <H2>Parameters and Dialog Box</H2>
      | <P>
      | <B>Output port width</B> this value must be specified, and must be the same as the associated value on the BKIN UDP Receieve Port Reset Block.
      | <P>
      | <B>Allow variable length packets: </B> This input is left-over from the legacy block. Leave unchecked, as it is has not been tested yet.
      | <P>
      | <B>Sample Time: </B> May be set to a faster update rate than the BKIN UDP Receive Port Reset.
      | <P>
      | 
      | <H2>Related Blocks </H2>
      | BKIN UDP Receive Port Reset<BR>
      mask Display:
      | disp( sprintf('BKIN UDP\nReceive\nBinary\n(%d bytes)', width));
      | port_label('output', 1, 'Data');
      | port_label('output', 2, 'N');
      | port_label('output', 3, 'Data 2');
      | port_label('output', 4, 'N 2');
      | port_label('output', 5, '# double reads');
      | port_label('output', 6, 'Request UDP Reset');
      | port_label('input', 1, 'UDP Reset Trigger');
      | port_label('input', 2, 'Port Info');
  UDP Receive Port Reset : S-Function  FunctionName=BKINUDPReceiveInit  Parameters=ipAdd, ipPort, width, sampletime, vblLen  mask(BKIN UDP Receive Port Reset){ipAddress=192.168.0.1, ipPort=50001, width=21, vblLen=off, sampletime=0.001}
      mask prompts: ipAddress "Source IP address:"; ipPort "Local (destination) port:"; width "Output port width (number of bytes):"; vblLen "Allow variable length packets"; sampletime "Sample time:"
      mask help:
      | Modified from legacy UDP Receive block.
      | The rationale for modifying was to enable resetting of the UDP Port while running a model.
      | Because resetting can potentially take longer than one clock cycle, the resetting needed to be split off from the reading to allow them to run at different update rates.
      |
      | Click Help for more details.
      mask init:
      | mudp('ipPort', 'IP Port');
      | ipAdd = ipAddressFromString(ipAddress);
      mask Help:
      | Used to read UDP packets. Modified from legacy UDP Read Receive. Must be used with BKIN UDP Receive Read block.
      | 
      | <H2>Description </H2>
      | This block initializes, closes, and can reset a UDP Receive port.
      | <P>
      | 
      | <B>UDP Reset: </B> this input must come from a BKIN UDP Receive Read block. When this input goes to 1, it will initiate a reset of the UDP port. It will send an acknowledgement that a reset is occuring as part of the output Port Info
      | <P>
      | <B># Resets: </B> This output contains the number of times that the UDP port has been reset.
      | <P>
      | <B>Port Info: </B> this vector output must go to the BKIN UDP Receive Read block. It contains information related to the port ID, the length of the expected packet and the status of the port reset.
      | <P>
      | 
      | <H2>Parameters and Dialog Box</H2>
      | <P>
      | <B>Source IP Address</B> in the form of xxx.xxx.xxx.xxx
      | <P>
      | <B>Local (destination) port</B> the port to be used.
      | <P>
      | <B>Output port width</B> this value must be specified, and must be the same as the associated value on the BKIN UDP Receieve Read Block.
      | <P>
      | <B>Sample time: </B> May be set to a slower update rate than the BKIN UDP Receive Read.
      | <P>
      | 
      | <H2>Related Blocks </H2>
      | BKIN UDP Receive Read<BR>
      mask Display:
      | disp( sprintf('BKIN UDP\nReceive\nPort Reset\n  (%d bytes)', width));
      | port_label('output', 1, '# Resets');
      | port_label('output', 2, 'Port Info');
      | port_label('input', 1, 'UDP Reset');
  Unpack : xpcobsoletelib/Utilities/Unpack   dimensions={[1]}  datatypes={'int32'}  byteAlign=1
  ACK_ID : Outport
  wires:
  Trigger UDP reset/1 -> Memory2/1
  Data Type Conversion/1 -> ACK_ID/1
  UDP Receive/2 -> Terminator7/1  "Pckt_Recd"
  UDP Receive/5 -> Terminator5/1  "# double reads"
  UDP Receive/6 -> Rate Transition1/1
  UDP Receive Port Reset/1 -> Terminator6/1  "# UDP Resets"
  Rate Transition1/1 -> UDP Receive Port Reset/1  "Rqst UDP Reset"
  Rate Transition2/1 -> UDP Receive/2
  Memory2/1 -> UDP Receive/1  "trigger"
  UDP Receive Port Reset/2 -> Memory1/1
  UDP Receive/3 -> Terminator3/1  "Data 2"
  UDP Receive/4 -> Terminator4/1  "Pckt_Recd 2"
  Unpack/1 -> Data Type Conversion/1
  Selector/1 -> Unpack/1
  UDP Receive/1 -> Selector/1
  Memory1/1 -> Rate Transition2/1

== system EMC_no_gaze/DataLogging/Network Transfer Subsystem/UDP Send Subsystem ==
  packet_data : Inport
  Trigger : TriggerPort  TriggerType=function-call
  Counter Free-Running : simulink/Sources/Counter Free-Running  NumBits=32  tsamp=-1
  Pack : xpcobsoletelib/Utilities/Pack   datatypes={'single'}  byteAlign=1
  Send : xpcrtudplib/Legacy UDP/Send   ipAddress=192.168.0.1  ipPort=50000  localPort=50000  vblLen=on  sampletime=-1
  Width : Width
  total_packets_sent : Outport  InitialOutput=0
  wires:
  Pack/1 -> Width/1, Send/1
  Counter Free-Running/1 -> total_packets_sent/1
  packet_data/1 -> Pack/1
  Width/1 -> Send/2

== system EMC_no_gaze/DataLogging/Network Transfer Subsystem/force strobe ==
  In1 : Inport
  Rate Transition1 : RateTransition  Integrity=off
  Rate Transition2 : RateTransition  Integrity=off
  force strobe : MATLAB Function  TreatAsAtomicUnit=on  SystemSampleTime=0.0005
  Out1 : Outport
  wires:
  Rate Transition2/1 -> Out1/1
  Rate Transition1/1 -> force strobe/1(strobe)
  In1/1 -> Rate Transition1/1
  force strobe/1(strobe_out) -> Rate Transition2/1

== system EMC_no_gaze/DataLogging/Poll Force Plates/plate1 ==
  gain : Inport
  calib_matrix : Inport  Port=2
  ain_slope : Inport  Port=3
  ain_offset : Inport  Port=4
  orientation : Inport  Port=5
  zero_voltage : Inport  Port=6
  Enable : EnablePort
  Receive : xpcrtudplib/Legacy UDP/Receive   ipAddress=192.168.0.101  ipPort=53795  width=64  vblLen=off  sampletime=BKIN_STEP_TIME
  Terminator : Terminator
  parse packet 1 : MATLAB Function  TreatAsAtomicUnit=on
  Forces P1 : Outport
  Moments P1 : Outport  Port=2
  Timer P1 : Outport  Port=3
  wires:
  parse packet 1/3(timer) -> Timer P1/1
  Receive/2 -> Terminator/1
  gain/1 -> parse packet 1/3(gain)
  Receive/1 -> parse packet 1/1(packet)
  calib_matrix/1 -> parse packet 1/2(calibration)
  parse packet 1/1(forces) -> Forces P1/1
  parse packet 1/2(moments) -> Moments P1/1
  ain_offset/1 -> parse packet 1/5(ain_offset)
  ain_slope/1 -> parse packet 1/4(ain_slope)
  orientation/1 -> parse packet 1/6(orientation)
  zero_voltage/1 -> parse packet 1/7(zero_voltage)

== system EMC_no_gaze/DataLogging/Poll Force Plates/plate2 ==
  gain : Inport
  calib_matrix : Inport  Port=2
  ain_slope : Inport  Port=3
  ain_offset : Inport  Port=4
  orientation : Inport  Port=5
  zero_voltage : Inport  Port=6
  Enable : EnablePort
  Receive1 : xpcrtudplib/Legacy UDP/Receive   ipAddress=192.168.0.102  ipPort=53796  width=64  vblLen=off  sampletime=BKIN_STEP_TIME
  Terminator : Terminator
  parse packet 1 : MATLAB Function  TreatAsAtomicUnit=on
  Forces P1 : Outport
  Moments P1 : Outport  Port=2
  Timer P1 : Outport  Port=3
  wires:
  parse packet 1/3(timer) -> Timer P1/1
  Receive1/2 -> Terminator/1
  gain/1 -> parse packet 1/3(gain)
  Receive1/1 -> parse packet 1/1(packet)
  calib_matrix/1 -> parse packet 1/2(calibration)
  parse packet 1/1(forces) -> Forces P1/1
  parse packet 1/2(moments) -> Moments P1/1
  ain_offset/1 -> parse packet 1/5(ain_offset)
  ain_slope/1 -> parse packet 1/4(ain_slope)
  orientation/1 -> parse packet 1/6(orientation)
  zero_voltage/1 -> parse packet 1/7(zero_voltage)

== system EMC_no_gaze/DataLogging/Poll Force Plates/send poll 1 ==
  send packet : Inport
  Enable : EnablePort
  Send : xpcrtudplib/Legacy UDP/Send   ipAddress=192.168.0.101  ipPort=52360  localPort=53795  vblLen=on  sampletime=0.0005
  Width : Width
  wires:
  Width/1 -> Send/2
  send packet/1 -> Send/1, Width/1

== system EMC_no_gaze/DataLogging/Poll Force Plates/send poll 2 ==
  send packet : Inport
  Enable : EnablePort
  Send1 : xpcrtudplib/Legacy UDP/Send   ipAddress=192.168.0.102  ipPort=52360  localPort=53796  vblLen=on  sampletime=0.0005
  Width : Width
  wires:
  Width/1 -> Send1/2
  send packet/1 -> Send1/1, Width/1

== system EMC_no_gaze/DataLogging/Poll KINARM/Force Sensor Control ==
  note: This subsystem receives data from force sensors in the KINARM setup, and starts and stops the data transfer in response to changes in
      | the force sensor parameters in the system above. Each KINARM EP can have a force sensor, so there can currently be up to two in a
      | given setup. The force sensors transmit data over UDP, and parameters of the data transfer (such as the data rate and IP address) are
      | configured for each force sensor individually via a web interface they provide. BKIN preconfigures force sensors with IP addresses
      | 192.168.0.10-11, where the first address is given to the sensor for robot 1 and the second to that for robot 2.
  note: Each subsystem also handles the receiving of data from its particular sensor. When a sensor is indicated as present, the latest data from
      | its IP is unpacked and placed into a 1x6 array (zeros are explicitly specified when a sensor is indicated as not present). The arrays for
      | the individual sensors are combined into a 2x6 matrix, similar to how robot data is handled in the system above.
      |
      | Each packet received from a force sensor contains the following:
      |      sequence number [uint32]
      |      internal sequence number [uint32]
      |      system status code [uint32]
      |      x-axis force [int32]
      |      y-axis force [int32]
      |      z-axis force [int32]
      |      x-axis torque [int32]
      |      y-axis torque [int32]
      |      z-axis torque [int32]
      |
      | For more information, again see the ATI Net Interface guide.
  note: Each "force sensor x" subsystem here starts and stops the data transfer from its respective force sensor. When the input flag indicating
      | the presence (1: yes, 0: no) of a force sensor changes, the respective subsystem sends a command message via UDP to that force
      | sensor's IP address that starts or stops the data transfer accordingly. For details about the structure of the command message, see the
      | ATI Net Interface guide.
      |
      | Note that the default setting for all force sensors is 1, for "present", in the system above. This is done so that whenever BKIN's client
      | software applies hardware settings to a task program, it must first lower all force sensor flags and then raise those for whichever sensors
      | are present again. This forces all sensors off in case they were not stopped properly by a previous task. This would not stop data that
      | had been transmitted from being received, so when a force sensor is marked as not present the data is zeroed explicitly.
  has FT : Inport
  Demux : Demux  Outputs=2
  Force Sensor 1 Subsystem : Subsystem
  Force Sensor 2 Subsystem : Subsystem
  Mux1 : Mux  Inputs=2
  Mux8 : Mux  Inputs=2
  Force Sensor Data : Outport
  Force Sensor Status : Outport  Port=2
  wires:
  Force Sensor 1 Subsystem/1(Out1) -> Mux8/1
  Force Sensor 2 Subsystem/1(Out1) -> Mux8/2
  has FT/1 -> Demux/1
  Demux/1 -> Force Sensor 1 Subsystem/1(Force Sensor 1 Present)
  Demux/2 -> Force Sensor 2 Subsystem/1(Force Sensor 2 Present)
  Mux8/1 -> Force Sensor Data/1
  Force Sensor 1 Subsystem/2(status) -> Mux1/1
  Force Sensor 2 Subsystem/2(status) -> Mux1/2
  Mux1/1 -> Force Sensor Status/1

== system EMC_no_gaze/DataLogging/Poll KINARM/PMAC Subsystem ==
  note: 1) replaced the variable 'orientation' with two variables: 'robot_orientation' and 'arm_orientation'.  Add comments to better explain.
      | 2) replaced the variables 'uncorrected_shoulder_angle' and 'uncorrected_elbow_angle' with 'relative_shoulder_angle' and 'relative_elbow_angle'
      | 3) replaced the variables corrected_shoulder_angle and corrected_elbow_angle with shoulder_angle and elbow_angle
      | 4) primary encoder data was not being corrected properly (for errors in non-perfect parallelogram structure) in the original.  This has now been fixed.
      | 5) replaced "if (robot_type < 1.0 && orientation == 2) || (robot_type > 0.0 && orientation == 1)"
      |             with "(robot_orientation == -1)"
  note: This block provides access to KINARM data for both BKIN client software and task program authors. Client software must provide
      | correct hardware information and calibration parameters for each KINARM, and this information is subsequently used to read
      | and scale data from the motion control card. The KINARM data and other attributes of the KINARM setup controlled by client
      | software, such as which arm is "dominant" for the KINARM EXO or EP, are combined into the KINdata structure. Arm kinematics
      | are output for inclusion in the current data frame.
      |
      | This block also offers client software access to the motion control card DPRAM via the DPRAM access subsystem.
      |
      | Note: The mask replaces the ZeroTorque constant with a From block that includes the commanded torques providing the model
      | includes an instance of the load-applying block.
      |
      | Note: For each Goto block created here, a corresponding From block is included in the Terminators for Gotos subsystem. This is
      | solely to prevent unnecessary warnings at the Matlab prompt if such From blocks are not present.
  enable : Inport
  run : Inport  Port=2
  pmac robot params : Inport  Port=3
  Bus Selector : BusSelector  OutputSignals=pmac robot1 params,pmac robot2 params
  read_pmac : Subsystem
      settings: RTWSystemCode=Nonreusable function  RTWFileNameOpts=Use function name
  update settings : Subsystem
  pmac force scale : Outport
  wires:
  read_pmac/1(robot data) -> update settings/1(Kinematics)
  read_pmac/2(servo counter) -> update settings/2(Servo counter)
  read_pmac/3(delay estimates) -> update settings/3(delay estimates)
  read_pmac/4(primary_encoder data) -> update settings/4(primry enc data)
  read_pmac/5(ep calibration bitfield) -> update settings/5(EP Calibration Button)
  read_pmac/6(status data) -> update settings/6(Robot status)
  run/1 -> update settings/Trigger
  enable/1 -> [enable]
  [enable] -> read_pmac/Enable
  pmac robot params/1 -> Bus Selector/1
  Bus Selector/1 -> read_pmac/1(pmac robot1 params)  "<pmac robot1 params>"
  Bus Selector/2 -> read_pmac/2(pmac robot2 params)  "<pmac robot2 params>"
  read_pmac/7(force scale) -> pmac force scale/1

== system EMC_no_gaze/DataLogging/Poll KINARM/bkin_internal_testing ==
  bkin_testing : Inport
  Data receive : Subsystem
  Data write : Subsystem
  ispmac1 : simulink/Logic and Bit Operations/Compare To Constant  relop===  const=3  OutDataTypeStr=boolean
  wires:
  bkin_testing/1 -> Data write/Trigger
  [system_type] -> ispmac1/1
  ispmac1/1 -> Data receive/Enable
  Data receive/3(servo counter) -> Data write/3(Servo counter)
  Data receive/4(EP calibration btn) -> Data write/4(EP Calibration Button)
  Data receive/5(Status bits) -> Data write/5(Robot status)
  Data receive/2(primary enc) -> Data write/2(primry enc data)
  Data receive/1(Kinematics) -> Data write/1(Kinematics)
